simulink model "EDS_Simulink_Model_02"  (R2022a)
settings: Solver=VariableStepAuto  StartTime=0.0  StopTime=stop_time  MaxStep=1e-5  RelTol=1e-3
values from neighbouring files (symbols this model uses):
  a = a/180*pi    [EDS_Script_Model_01.m]    (also in EDS_Script_Model_02.m)
  accel = wheel_radps/accel_time    [EDS_Script_Model_01.m]    (also in EDS_Script_Model_02.m)
  accel_time = 5.33    [EDS_Script_Model_01.m]    (also in EDS_Script_Model_02.m)
  Cx = 0.25    [EDS_Script_Model_01.m]    (also in EDS_Script_Model_02.m)
  d = 1.5    [EDS_Script_Model_01.m]    (also in EDS_Script_Model_02.m)
  density = 1.3    [EDS_Script_Model_01.m]    (also in EDS_Script_Model_02.m)
  F = 4e-04    (= 0.0004)    [EDS_Script_Model_02.m]
  Filter_coefficient = 100/50    (= 2)    [EDS_Script_Model_02.m]
  fr = 0.01    [EDS_Script_Model_01.m]    (also in EDS_Script_Model_02.m)
  g = 9.81    [EDS_Script_Model_01.m]    (also in EDS_Script_Model_02.m)
  i_gear = 7.2    [EDS_Script_Model_01.m]    (also in EDS_Script_Model_02.m = 1)
  J = 0.07/4    (= 0.0175)    [EDS_Script_Model_02.m]
  K_tor_all_1 = 1/2    (= 0.5)    [EDS_Script_Model_01.m]    (also in EDS_Script_Model_02.m)
  K_tor_all_2 = 1/2    (= 0.5)    [EDS_Script_Model_01.m]    (also in EDS_Script_Model_02.m)
  Kd_w = 0.5/8    (= 0.0625)    [EDS_Script_Model_02.m]
  Ki_id = 0.2/14    (= 0.0142857142857)    [EDS_Script_Model_02.m]
  Ki_iq = 10/14    (= 0.714285714286)    [EDS_Script_Model_02.m]
  Ki_w = 2/0.024    (= 83.3333333333)    [EDS_Script_Model_02.m]
  Kp_id = 5/12    (= 0.416666666667)    [EDS_Script_Model_02.m]
  Kp_iq = 30/12    (= 2.5)    [EDS_Script_Model_02.m]
  Kp_w = 55/0.024    (= 2291.66666667)    [EDS_Script_Model_02.m]
  L = 2.5    [EDS_Script_Model_01.m]    (also in EDS_Script_Model_02.m)
  M = 1200    [EDS_Script_Model_01.m]    (also in EDS_Script_Model_02.m)
  n_eff_gear = 0.98    [EDS_Script_Model_01.m]    (also in EDS_Script_Model_02.m = 1)
  p = 4    [EDS_Script_Model_02.m]
  Rs = 4.47-1.47-0.40    (= 2.6)    [EDS_Script_Model_02.m]
  Rw = 0.26    [EDS_Script_Model_01.m]    (also in EDS_Script_Model_02.m)
  S = 1.9    [EDS_Script_Model_01.m]    (also in EDS_Script_Model_02.m)
  Satur_max_PI_id = Vdc_1*sqrt(1/3)    [EDS_Script_Model_02.m]
  Satur_max_PI_iq = Vdc_1*sqrt(1/3)    [EDS_Script_Model_02.m]
  Satur_max_PI_w = 40+30    (= 70)    [EDS_Script_Model_02.m]
  Satur_min_PI_id = -Vdc_1*sqrt(1/3)    [EDS_Script_Model_02.m]
  Satur_min_PI_iq = -Vdc_1*sqrt(1/3)    [EDS_Script_Model_02.m]
  Satur_min_PI_w = -40-30    (= -70)    [EDS_Script_Model_02.m]
  steering_angle_1 = steering_angle_1_m(ii)    [EDS_Script_Model_01.m]    (also in EDS_Script_Model_02.m)
  steering_angle_2 = steering_angle_2_m(ii)    [EDS_Script_Model_01.m]    (also in EDS_Script_Model_02.m)
  steering_angle_3 = steering_angle_3_m(ii)    [EDS_Script_Model_01.m]    (also in EDS_Script_Model_02.m)
  steering_angle_4 = steering_angle_4_m(ii)    [EDS_Script_Model_01.m]    (also in EDS_Script_Model_02.m)
  steering_angle_initial = steering_angle_initial_m(ii)    [EDS_Script_Model_01.m]    (also in EDS_Script_Model_02.m)
  Tf = 0    [EDS_Script_Model_02.m]
  time_steering_angle_1 = 8    [EDS_Script_Model_01.m]    (also in EDS_Script_Model_02.m)
  time_steering_angle_2 = 10    [EDS_Script_Model_01.m]    (also in EDS_Script_Model_02.m)
  time_steering_angle_3 = 14    [EDS_Script_Model_01.m]    (also in EDS_Script_Model_02.m)
  time_steering_angle_4 = 18    [EDS_Script_Model_01.m]    (also in EDS_Script_Model_02.m)
  Vdc_1 = 500    [EDS_Script_Model_02.m]
  Vdc_2 = 500    [EDS_Script_Model_02.m]
  Vf = 0    [EDS_Script_Model_02.m]
  Vfd = 0    [EDS_Script_Model_02.m]
undefined symbols (not defined in the file or in its folder): time_w_ref_1, time_w_ref_2, w_ref_1, w_ref_2, w_ref_initial
libraries: slpidlib x6, spsPermanentMagnetSynchronousMachineLib x2, spsThreePhaseVIMeasurementLib x2, spsUniversalBridgeLib x2, spsDCVoltageSourceLib x2, spsVoltageMeasurementLib x2, spspowerguiLib x1
(part 1 of 2)
settings Model: Creator=panos  LastModifiedBy=panos
settings SolverCC: ConsecutiveZCsStepRelTol=128*eps  MaxConsecutiveZCs=5000
settings DataIOCC: MaxDataPoints=5e5  Refine=4
settings DebuggingCC: IgnoredZcDiagnostic=none

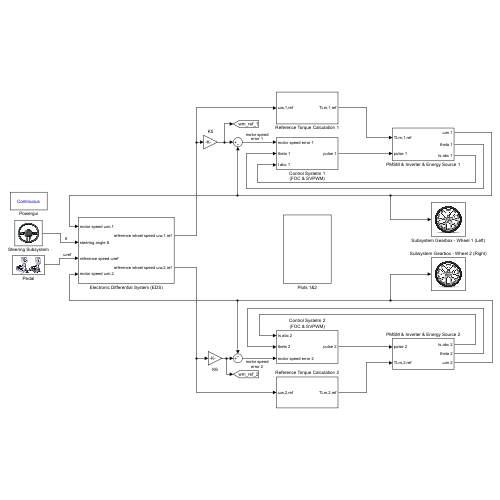
[thumbnail: Simulink's stored preview of the top-level diagram]
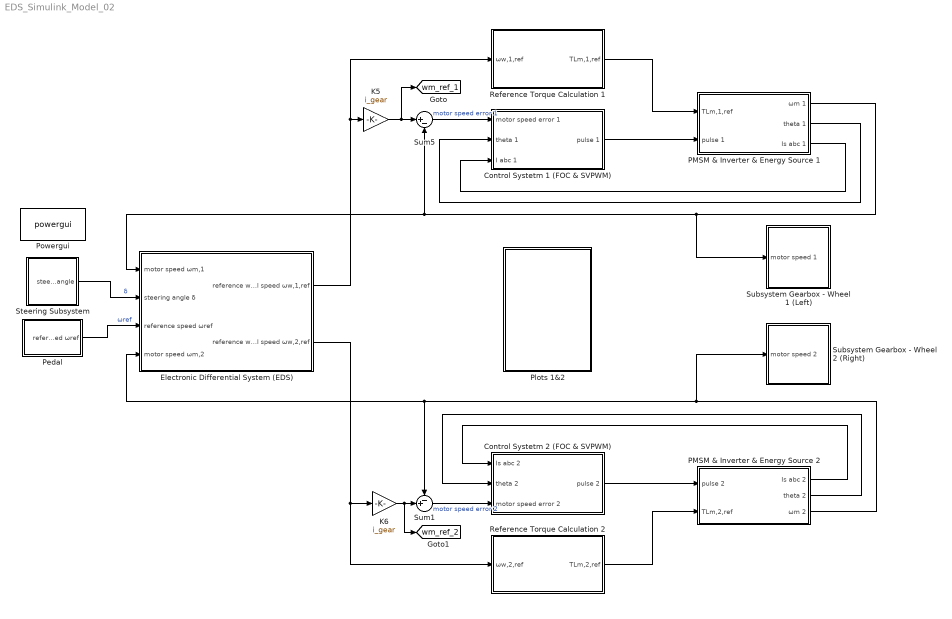
== system EDS_Simulink_Model_02 ==
  Control Systetm 1 (FOC & SVPWM) : Subsystem
  Control Systetm 2 (FOC & SVPWM) : Subsystem
  Electronic Differential System (EDS) : Subsystem
  K5 : Gain  Gain=i_gear
  K6 : Gain  Gain=i_gear
  PMSM & Inverter & Energy Source 1 : Subsystem
  PMSM & Inverter & Energy Source 2 : Subsystem
  Pedal : Subsystem
      mask Display: image('pedal.jpg'); % Use "Edit Image" on toolstrip to change.
  Plots 1&2 : Subsystem
  Powergui : spspowerguiLib/powergui  Priority=1  SimulationMode=Continuous  SampleTime=50e-6  frequency=60  Iterations=50  frequencyindice=0  Pbase=100e6  ErrMax=1e-4  UnitsV=kV  UnitsW=MW  buscounter=0  FunctionMessages=off  echomessages=off  EnableUseOfTLC=off  CurrentSourceSwitches=off  DisableSnubberDevices=off  DisableRonSwitches=off  DisableVfSwitches=off  DisplayEquations=off  AutomaticDiscreteSolvers=off  SolverType=Tustin/Backward Euler (TBE)  Interpol=off  ExternalGateDelay=off  methode=off  Ts=100  x0status=blocks  SPID=on  SwTol=0  HookPort=off  NonlinearTolerance=1e-4  nMaxIteration=100  ContinueOnMaxIteration=off  RestoreLinks=warning  ResistiveCurrentMeasurement=off  Frange=[0:2:500]  Ylog=off  Xlog=on  ShowGrid=off  save=off  variable=ZData  structure=0  ZoomFFT=off  StartTime=0.0  cycles=1  DisplayStyle=1  fundamental=60  FreqAxis=off  MaxFrequency=1000  frequencyindicesteady=1  RmsSteady=1  display=off
  Reference Torque Calculation 1 : Subsystem
  Reference Torque Calculation 2 : Subsystem
  Steering Subsystem : Subsystem
      mask Display: image('steering.jpg'); % Use "Edit Image" on toolstrip to change.
  Subsystem Gearbox - Wheel 1 (Left) : Subsystem
      mask Display: image('C:\Users\panos\OneDrive\Υπολογιστής\Desktop\Master_Thesis\electronic differential system (EDS)\PHOTO\wheel.jpg'); % Use "Edit Image" on toolstrip to change.
  Subsystem Gearbox - Wheel 2 (Right) : Subsystem
      mask Display: image('C:\Users\panos\OneDrive\Υπολογιστής\Desktop\Master_Thesis\electronic differential system (EDS)\PHOTO\wheel.jpg'); % Use "Edit Image" on toolstrip to change.
  Sum1 : Sum  Inputs=-+|
  Sum5 : Sum  Inputs=|+-
  tag scope: wm_ref_1=global, wm_ref_2=global
  wires:
  Sum1/1 -> Control Systetm 2 (FOC & SVPWM)/3(motor speed error 2)  "motor speed error 2"
  PMSM & Inverter & Energy Source 2/3(ωm 2) -> Sum1/1, Electronic Differential System (EDS)/4(motor speed ωm,2), Subsystem Gearbox - Wheel 2 (Right)/1(motor speed 2)
  Sum5/1 -> Control Systetm 1 (FOC & SVPWM)/1(motor speed error 1)  "motor speed error 1"
  PMSM & Inverter & Energy Source 1/1(ωm 1) -> Subsystem Gearbox - Wheel 1 (Left)/1(motor speed 1), Sum5/2, Electronic Differential System (EDS)/1(motor speed ωm,1)
  Electronic Differential System (EDS)/1("reference wheel speed ωw,1,ref ") -> Reference Torque Calculation 1/1(ωw,1,ref), K5/1
  Electronic Differential System (EDS)/2("reference wheel speed ωw,2,ref ") -> Reference Torque Calculation 2/1(ωw,2,ref), K6/1
  Steering Subsystem/1(steering angle) -> Electronic Differential System (EDS)/2(steering angle δ)  "δ"
  Pedal/1(reference speed ωref) -> Electronic Differential System (EDS)/3(reference speed ωref)  "ωref"
  Reference Torque Calculation 1/1(TLm,1,ref) -> PMSM & Inverter & Energy Source 1/1(TLm,1,ref)
  Reference Torque Calculation 2/1(TLm,2,ref) -> PMSM & Inverter & Energy Source 2/2(TLm,2,ref)
  K6/1 -> Sum1/2, [wm_ref_2]
  Control Systetm 2 (FOC & SVPWM)/1(pulse 2) -> PMSM & Inverter & Energy Source 2/1(pulse 2)
  Control Systetm 1 (FOC & SVPWM)/1(pulse 1) -> PMSM & Inverter & Energy Source 1/2(pulse 1)
  PMSM & Inverter & Energy Source 1/2(theta 1) -> Control Systetm 1 (FOC & SVPWM)/2(theta 1)
  PMSM & Inverter & Energy Source 1/3(Is abc 1) -> Control Systetm 1 (FOC & SVPWM)/3(I abc 1)
  K5/1 -> [wm_ref_1], Sum5/1
  PMSM & Inverter & Energy Source 2/2(theta 2) -> Control Systetm 2 (FOC & SVPWM)/2(theta 2)
  PMSM & Inverter & Energy Source 2/1(Is abc 2) -> Control Systetm 2 (FOC & SVPWM)/1(Is abc 2)

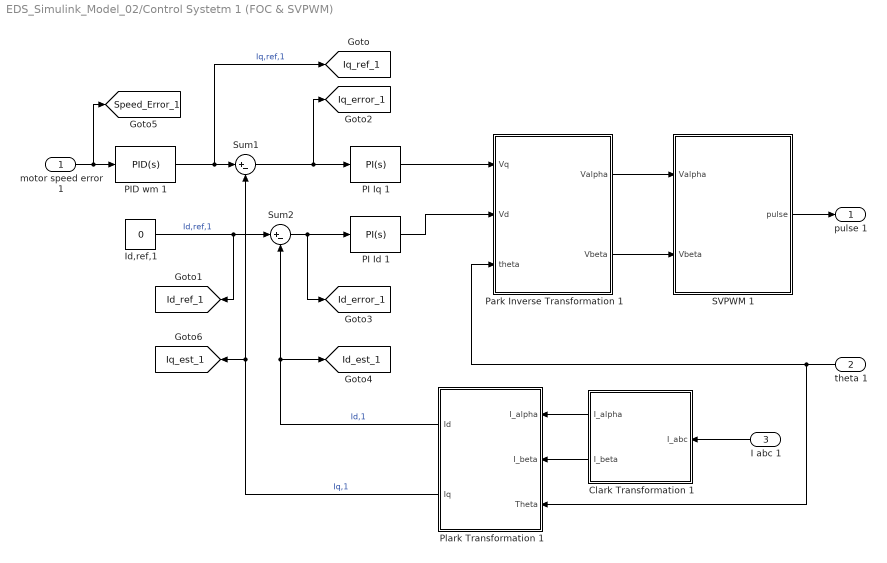
== system EDS_Simulink_Model_02/Control Systetm 1 (FOC & SVPWM) ==
  motor speed error 1 : Inport
  theta 1 : Inport  Port=2
  I abc 1 : Inport  Port=3
  Clark Transformation 1 : Subsystem
  Id,ref,1 : Constant  Value=0
  "PI Id 1 " : slpidlib/PID Controller  Controller=PI  Form=Parallel  TimeDomain=Continuous-time  UseExternalTs=off  SampleTime=-1  IntegratorMethod=Forward Euler  FilterMethod=Forward Euler  ControllerParametersSource=internal  P=Kp_id  I=Ki_id  UseKiTs=off  D=0  N=100  UseFilter=on  TunerSelectOption=Transfer Function Based (PID Tuner App)  InitialConditionSource=internal  InitialConditionForIntegrator=0  InitialConditionForFilter=0  DifferentiatorICPrevScaledInput=0  ExternalReset=none  TrackingMode=off  Kt=1  LimitOutput=on  SatLimitsSource=internal  UpperSaturationLimit=Satur_max_PI_id  LowerSaturationLimit=Satur_min_PI_id  LinearizeAsGain=on  AntiWindupMode=none  Kb=1  POutMin=[]  POutMax=[]  IOutMin=[]  IOutMax=[]  DOutMin=[]  DOutMax=[]  NOutMin=[]  NOutMax=[]  SumOutMin=[]  SumOutMax=[]  SaturationOutMin=[]  SaturationOutMax=[]  PParamMin=[]  PParamMax=[]  IParamMin=[]  IParamMax=[]  DParamMin=[]  DParamMax=[]  NParamMin=[]  NParamMax=[]  KbParamMin=[]  KbParamMax=[]  KtParamMin=[]  KtParamMax=[]  KbOutMin=[]  KbOutMax=[]  KtOutMin=[]  KtOutMax=[]  IntegratorOutMin=[]  IntegratorOutMax=[]  FilterOutMin=[]  FilterOutMax=[]  SumI1OutMin=[]  SumI1OutMax=[]  SumI2OutMin=[]  SumI2OutMax=[]  SumI3OutMin=[]  SumI3OutMax=[]  SumI4OutMin=[]  SumI4OutMax=[]  SumDOutMin=[]  SumDOutMax=[]  DifferentiatorOutMin=[]  DifferentiatorOutMax=[]  FilterDiffOutCoefMin=[]  FilterDiffOutCoefMax=[]  ReciprocalOutMin=[]  ReciprocalOutMax=[]  SumDenOutMin=[]  SumDenOutMax=[]  SumNumOutMin=[]  SumNumOutMax=[]  DivideOutMin=[]  DivideOutMax=[]  UdiffTsProdOutMin=[]  UdiffTsProdOutMax=[]  NTsProdOutMin=[]  NTsProdOutMax=[]  UintegralTsProdOutMin=[]  UintegralTsProdOutMax=[]  UngainTsProdOutMin=[]  UngainTsProdOutMax=[]  IntegratorContinuousStateAttributes=''  IntegratorStateMustResolveToSignalObject=off  IntegratorRTWStateStorageClass=Auto  FilterContinuousStateAttributes=''  FilterStateMustResolveToSignalObject=off  FilterRTWStateStorageClass=Auto  ParallelPVariant=InternalParameters  IdealPVariant=Disabled  IVariant=InternalParameters  DVariant=Disabled  IntegratorVariant=Continuous  SatVariant=Enabled  AWVariant=Passthrough  PCopyVariant=Disabled  TRVariant=Disabled  FdbkBlocksVariant=Forward  IdealPFdbkVariant=Disabled  SatFdbkVariant=Disabled  DerivativeFilterVariant=Disabled  NVariant=Disabled  NCopyVariant=Disabled_SignalSpec  FilterICVariant=Disabled  IntegratorICVariant=InternalICs  ExternalResetVariant=Disabled  TRSumVariant=Passthrough  SumFdbkVariant=Disabled  SumVariant=Sum_PI  TsampFilterVariant=InternalTs  TsampNgainVariant=Passthrough  TsampIntegralVariant=Passthrough  ExternalSaturationOutDataTypeStr=Inherit: Same as second input  aMode=0
  PI Iq 1 : slpidlib/PID Controller  Controller=PI  Form=Parallel  TimeDomain=Continuous-time  UseExternalTs=off  SampleTime=-1  IntegratorMethod=Forward Euler  FilterMethod=Forward Euler  ControllerParametersSource=internal  P=Kp_iq  I=Ki_iq  UseKiTs=off  D=0  N=100  UseFilter=on  TunerSelectOption=Transfer Function Based (PID Tuner App)  InitialConditionSource=internal  InitialConditionForIntegrator=0  InitialConditionForFilter=0  DifferentiatorICPrevScaledInput=0  ExternalReset=none  TrackingMode=off  Kt=1  LimitOutput=on  SatLimitsSource=internal  UpperSaturationLimit=Satur_max_PI_iq  LowerSaturationLimit=Satur_min_PI_iq  LinearizeAsGain=on  AntiWindupMode=none  Kb=1  POutMin=[]  POutMax=[]  IOutMin=[]  IOutMax=[]  DOutMin=[]  DOutMax=[]  NOutMin=[]  NOutMax=[]  SumOutMin=[]  SumOutMax=[]  SaturationOutMin=[]  SaturationOutMax=[]  PParamMin=[]  PParamMax=[]  IParamMin=[]  IParamMax=[]  DParamMin=[]  DParamMax=[]  NParamMin=[]  NParamMax=[]  KbParamMin=[]  KbParamMax=[]  KtParamMin=[]  KtParamMax=[]  KbOutMin=[]  KbOutMax=[]  KtOutMin=[]  KtOutMax=[]  IntegratorOutMin=[]  IntegratorOutMax=[]  FilterOutMin=[]  FilterOutMax=[]  SumI1OutMin=[]  SumI1OutMax=[]  SumI2OutMin=[]  SumI2OutMax=[]  SumI3OutMin=[]  SumI3OutMax=[]  SumI4OutMin=[]  SumI4OutMax=[]  SumDOutMin=[]  SumDOutMax=[]  DifferentiatorOutMin=[]  DifferentiatorOutMax=[]  FilterDiffOutCoefMin=[]  FilterDiffOutCoefMax=[]  ReciprocalOutMin=[]  ReciprocalOutMax=[]  SumDenOutMin=[]  SumDenOutMax=[]  SumNumOutMin=[]  SumNumOutMax=[]  DivideOutMin=[]  DivideOutMax=[]  UdiffTsProdOutMin=[]  UdiffTsProdOutMax=[]  NTsProdOutMin=[]  NTsProdOutMax=[]  UintegralTsProdOutMin=[]  UintegralTsProdOutMax=[]  UngainTsProdOutMin=[]  UngainTsProdOutMax=[]  IntegratorContinuousStateAttributes=''  IntegratorStateMustResolveToSignalObject=off  IntegratorRTWStateStorageClass=Auto  FilterContinuousStateAttributes=''  FilterStateMustResolveToSignalObject=off  FilterRTWStateStorageClass=Auto  ParallelPVariant=InternalParameters  IdealPVariant=Disabled  IVariant=InternalParameters  DVariant=Disabled  IntegratorVariant=Continuous  SatVariant=Enabled  AWVariant=Passthrough  PCopyVariant=Disabled  TRVariant=Disabled  FdbkBlocksVariant=Forward  IdealPFdbkVariant=Disabled  SatFdbkVariant=Disabled  DerivativeFilterVariant=Disabled  NVariant=Disabled  NCopyVariant=Disabled_SignalSpec  FilterICVariant=Disabled  IntegratorICVariant=InternalICs  ExternalResetVariant=Disabled  TRSumVariant=Passthrough  SumFdbkVariant=Disabled  SumVariant=Sum_PI  TsampFilterVariant=InternalTs  TsampNgainVariant=Passthrough  TsampIntegralVariant=Passthrough  ExternalSaturationOutDataTypeStr=Inherit: Same as second input  aMode=0
  PID wm 1 : slpidlib/PID Controller  Controller=PID  Form=Parallel  TimeDomain=Continuous-time  UseExternalTs=off  SampleTime=-1  IntegratorMethod=Forward Euler  FilterMethod=Forward Euler  ControllerParametersSource=internal  P=Kp_w  I=Ki_w  UseKiTs=off  D=Kd_w  N=Filter_coefficient  UseFilter=on  TunerSelectOption=Transfer Function Based (PID Tuner App)  InitialConditionSource=internal  InitialConditionForIntegrator=0  InitialConditionForFilter=0  DifferentiatorICPrevScaledInput=0  ExternalReset=none  TrackingMode=off  Kt=1  LimitOutput=on  SatLimitsSource=internal  UpperSaturationLimit=Satur_max_PI_w  LowerSaturationLimit=Satur_min_PI_w  LinearizeAsGain=on  AntiWindupMode=none  Kb=1  POutMin=[]  POutMax=[]  IOutMin=[]  IOutMax=[]  DOutMin=[]  DOutMax=[]  NOutMin=[]  NOutMax=[]  SumOutMin=[]  SumOutMax=[]  SaturationOutMin=[]  SaturationOutMax=[]  PParamMin=[]  PParamMax=[]  IParamMin=[]  IParamMax=[]  DParamMin=[]  DParamMax=[]  NParamMin=[]  NParamMax=[]  KbParamMin=[]  KbParamMax=[]  KtParamMin=[]  KtParamMax=[]  KbOutMin=[]  KbOutMax=[]  KtOutMin=[]  KtOutMax=[]  IntegratorOutMin=[]  IntegratorOutMax=[]  FilterOutMin=[]  FilterOutMax=[]  SumI1OutMin=[]  SumI1OutMax=[]  SumI2OutMin=[]  SumI2OutMax=[]  SumI3OutMin=[]  SumI3OutMax=[]  SumI4OutMin=[]  SumI4OutMax=[]  SumDOutMin=[]  SumDOutMax=[]  DifferentiatorOutMin=[]  DifferentiatorOutMax=[]  FilterDiffOutCoefMin=[]  FilterDiffOutCoefMax=[]  ReciprocalOutMin=[]  ReciprocalOutMax=[]  SumDenOutMin=[]  SumDenOutMax=[]  SumNumOutMin=[]  SumNumOutMax=[]  DivideOutMin=[]  DivideOutMax=[]  UdiffTsProdOutMin=[]  UdiffTsProdOutMax=[]  NTsProdOutMin=[]  NTsProdOutMax=[]  UintegralTsProdOutMin=[]  UintegralTsProdOutMax=[]  UngainTsProdOutMin=[]  UngainTsProdOutMax=[]  IntegratorContinuousStateAttributes=''  IntegratorStateMustResolveToSignalObject=off  IntegratorRTWStateStorageClass=Auto  FilterContinuousStateAttributes=''  FilterStateMustResolveToSignalObject=off  FilterRTWStateStorageClass=Auto  ParallelPVariant=InternalParameters  IdealPVariant=Disabled  IVariant=InternalParameters  DVariant=InternalParameters  IntegratorVariant=Continuous  SatVariant=Enabled  AWVariant=Passthrough  PCopyVariant=Disabled  TRVariant=Disabled  FdbkBlocksVariant=Forward  IdealPFdbkVariant=Disabled  SatFdbkVariant=Disabled  DerivativeFilterVariant=ContFilter  NVariant=InternalParameters  NCopyVariant=Disabled  FilterICVariant=InternalICsFilter  IntegratorICVariant=InternalICs  ExternalResetVariant=Disabled  TRSumVariant=Passthrough  SumFdbkVariant=Disabled  SumVariant=Sum_PID  TsampFilterVariant=InternalTs  TsampNgainVariant=Passthrough  TsampIntegralVariant=Passthrough  ExternalSaturationOutDataTypeStr=Inherit: Same as second input  aMode=0
  "Park Inverse Transformation 1 " : Subsystem
  Plark Transformation 1 : Subsystem
  SVPWM 1 : Subsystem
  Sum1 : Sum  Inputs=|+-
  Sum2 : Sum  Inputs=|+-
  pulse 1 : Outport
  tag scope: Id_error_1=global, Id_est_1=global, Id_ref_1=global, Iq_error_1=global, Iq_est_1=global, Iq_ref_1=global, Speed_Error_1=global
  wires:
  PI Iq 1/1 -> "Park Inverse Transformation 1 "/1(Vq)
  PID wm 1/1 -> [Iq_ref_1], Sum1/1  "Iq,ref,1"
  "PI Id 1 "/1 -> "Park Inverse Transformation 1 "/2(Vd)
  Id,ref,1/1 -> Sum2/1, [Id_ref_1]  "Id,ref,1"
  Plark Transformation 1/2(Iq) -> [Iq_est_1], Sum1/2  "Iq,1"
  "Park Inverse Transformation 1 "/2(Vbeta) -> SVPWM 1/2(Vbeta)
  Clark Transformation 1/2(I_beta) -> Plark Transformation 1/2(I_beta)
  Plark Transformation 1/1(Id) -> Sum2/2, [Id_est_1]  "Id,1"
  Sum2/1 -> [Id_error_1], "PI Id 1 "/1
  theta 1/1 -> Plark Transformation 1/3(Theta), "Park Inverse Transformation 1 "/3(theta)
  "Park Inverse Transformation 1 "/1(Valpha) -> SVPWM 1/1(Valpha)
  I abc 1/1 -> Clark Transformation 1/1(I_abc)
  SVPWM 1/1(pulse) -> pulse 1/1
  Sum1/1 -> PI Iq 1/1, [Iq_error_1]
  motor speed error 1/1 -> PID wm 1/1, [Speed_Error_1]
  Clark Transformation 1/1(I_alpha) -> Plark Transformation 1/1(I_alpha)

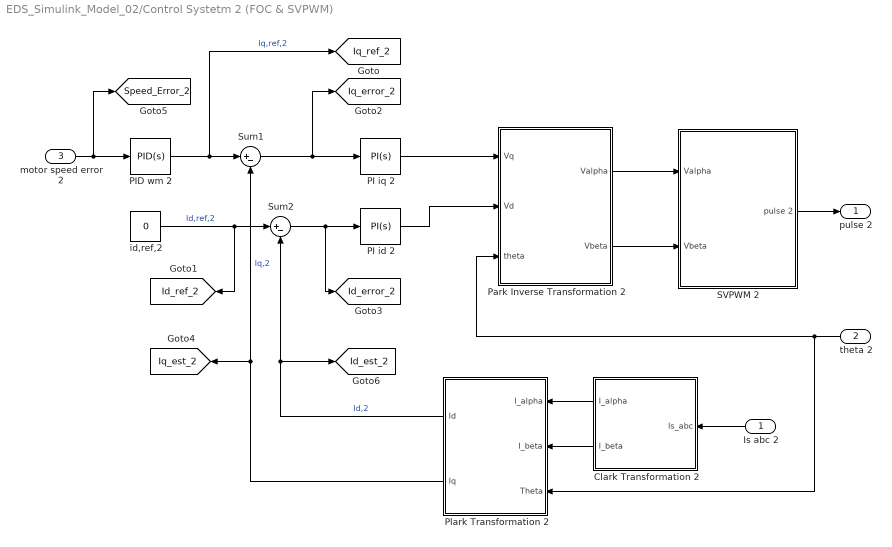
== system EDS_Simulink_Model_02/Control Systetm 2 (FOC & SVPWM) ==
  Is abc 2 : Inport
  theta 2 : Inport  Port=2
  motor speed error 2 : Inport  Port=3
  Clark Transformation 2 : Subsystem
  "PI id 2 " : slpidlib/PID Controller  Controller=PI  Form=Parallel  TimeDomain=Continuous-time  UseExternalTs=off  SampleTime=-1  IntegratorMethod=Forward Euler  FilterMethod=Forward Euler  ControllerParametersSource=internal  P=Kp_id  I=Ki_id  UseKiTs=off  D=0  N=100  UseFilter=on  TunerSelectOption=Transfer Function Based (PID Tuner App)  InitialConditionSource=internal  InitialConditionForIntegrator=0  InitialConditionForFilter=0  DifferentiatorICPrevScaledInput=0  ExternalReset=none  TrackingMode=off  Kt=1  LimitOutput=on  SatLimitsSource=internal  UpperSaturationLimit=Satur_max_PI_id  LowerSaturationLimit=Satur_min_PI_id  LinearizeAsGain=on  AntiWindupMode=none  Kb=1  POutMin=[]  POutMax=[]  IOutMin=[]  IOutMax=[]  DOutMin=[]  DOutMax=[]  NOutMin=[]  NOutMax=[]  SumOutMin=[]  SumOutMax=[]  SaturationOutMin=[]  SaturationOutMax=[]  PParamMin=[]  PParamMax=[]  IParamMin=[]  IParamMax=[]  DParamMin=[]  DParamMax=[]  NParamMin=[]  NParamMax=[]  KbParamMin=[]  KbParamMax=[]  KtParamMin=[]  KtParamMax=[]  KbOutMin=[]  KbOutMax=[]  KtOutMin=[]  KtOutMax=[]  IntegratorOutMin=[]  IntegratorOutMax=[]  FilterOutMin=[]  FilterOutMax=[]  SumI1OutMin=[]  SumI1OutMax=[]  SumI2OutMin=[]  SumI2OutMax=[]  SumI3OutMin=[]  SumI3OutMax=[]  SumI4OutMin=[]  SumI4OutMax=[]  SumDOutMin=[]  SumDOutMax=[]  DifferentiatorOutMin=[]  DifferentiatorOutMax=[]  FilterDiffOutCoefMin=[]  FilterDiffOutCoefMax=[]  ReciprocalOutMin=[]  ReciprocalOutMax=[]  SumDenOutMin=[]  SumDenOutMax=[]  SumNumOutMin=[]  SumNumOutMax=[]  DivideOutMin=[]  DivideOutMax=[]  UdiffTsProdOutMin=[]  UdiffTsProdOutMax=[]  NTsProdOutMin=[]  NTsProdOutMax=[]  UintegralTsProdOutMin=[]  UintegralTsProdOutMax=[]  UngainTsProdOutMin=[]  UngainTsProdOutMax=[]  IntegratorContinuousStateAttributes=''  IntegratorStateMustResolveToSignalObject=off  IntegratorRTWStateStorageClass=Auto  FilterContinuousStateAttributes=''  FilterStateMustResolveToSignalObject=off  FilterRTWStateStorageClass=Auto  ParallelPVariant=InternalParameters  IdealPVariant=Disabled  IVariant=InternalParameters  DVariant=Disabled  IntegratorVariant=Continuous  SatVariant=Enabled  AWVariant=Passthrough  PCopyVariant=Disabled  TRVariant=Disabled  FdbkBlocksVariant=Forward  IdealPFdbkVariant=Disabled  SatFdbkVariant=Disabled  DerivativeFilterVariant=Disabled  NVariant=Disabled  NCopyVariant=Disabled_SignalSpec  FilterICVariant=Disabled  IntegratorICVariant=InternalICs  ExternalResetVariant=Disabled  TRSumVariant=Passthrough  SumFdbkVariant=Disabled  SumVariant=Sum_PI  TsampFilterVariant=InternalTs  TsampNgainVariant=Passthrough  TsampIntegralVariant=Passthrough  ExternalSaturationOutDataTypeStr=Inherit: Same as second input  aMode=0
  PI iq 2 : slpidlib/PID Controller  Controller=PI  Form=Parallel  TimeDomain=Continuous-time  UseExternalTs=off  SampleTime=-1  IntegratorMethod=Forward Euler  FilterMethod=Forward Euler  ControllerParametersSource=internal  P=Kp_iq  I=Ki_iq  UseKiTs=off  D=0  N=100  UseFilter=on  TunerSelectOption=Transfer Function Based (PID Tuner App)  InitialConditionSource=internal  InitialConditionForIntegrator=0  InitialConditionForFilter=0  DifferentiatorICPrevScaledInput=0  ExternalReset=none  TrackingMode=off  Kt=1  LimitOutput=on  SatLimitsSource=internal  UpperSaturationLimit=Satur_max_PI_iq  LowerSaturationLimit=Satur_min_PI_iq  LinearizeAsGain=on  AntiWindupMode=none  Kb=1  POutMin=[]  POutMax=[]  IOutMin=[]  IOutMax=[]  DOutMin=[]  DOutMax=[]  NOutMin=[]  NOutMax=[]  SumOutMin=[]  SumOutMax=[]  SaturationOutMin=[]  SaturationOutMax=[]  PParamMin=[]  PParamMax=[]  IParamMin=[]  IParamMax=[]  DParamMin=[]  DParamMax=[]  NParamMin=[]  NParamMax=[]  KbParamMin=[]  KbParamMax=[]  KtParamMin=[]  KtParamMax=[]  KbOutMin=[]  KbOutMax=[]  KtOutMin=[]  KtOutMax=[]  IntegratorOutMin=[]  IntegratorOutMax=[]  FilterOutMin=[]  FilterOutMax=[]  SumI1OutMin=[]  SumI1OutMax=[]  SumI2OutMin=[]  SumI2OutMax=[]  SumI3OutMin=[]  SumI3OutMax=[]  SumI4OutMin=[]  SumI4OutMax=[]  SumDOutMin=[]  SumDOutMax=[]  DifferentiatorOutMin=[]  DifferentiatorOutMax=[]  FilterDiffOutCoefMin=[]  FilterDiffOutCoefMax=[]  ReciprocalOutMin=[]  ReciprocalOutMax=[]  SumDenOutMin=[]  SumDenOutMax=[]  SumNumOutMin=[]  SumNumOutMax=[]  DivideOutMin=[]  DivideOutMax=[]  UdiffTsProdOutMin=[]  UdiffTsProdOutMax=[]  NTsProdOutMin=[]  NTsProdOutMax=[]  UintegralTsProdOutMin=[]  UintegralTsProdOutMax=[]  UngainTsProdOutMin=[]  UngainTsProdOutMax=[]  IntegratorContinuousStateAttributes=''  IntegratorStateMustResolveToSignalObject=off  IntegratorRTWStateStorageClass=Auto  FilterContinuousStateAttributes=''  FilterStateMustResolveToSignalObject=off  FilterRTWStateStorageClass=Auto  ParallelPVariant=InternalParameters  IdealPVariant=Disabled  IVariant=InternalParameters  DVariant=Disabled  IntegratorVariant=Continuous  SatVariant=Enabled  AWVariant=Passthrough  PCopyVariant=Disabled  TRVariant=Disabled  FdbkBlocksVariant=Forward  IdealPFdbkVariant=Disabled  SatFdbkVariant=Disabled  DerivativeFilterVariant=Disabled  NVariant=Disabled  NCopyVariant=Disabled_SignalSpec  FilterICVariant=Disabled  IntegratorICVariant=InternalICs  ExternalResetVariant=Disabled  TRSumVariant=Passthrough  SumFdbkVariant=Disabled  SumVariant=Sum_PI  TsampFilterVariant=InternalTs  TsampNgainVariant=Passthrough  TsampIntegralVariant=Passthrough  ExternalSaturationOutDataTypeStr=Inherit: Same as second input  aMode=0
  PID wm 2 : slpidlib/PID Controller  Controller=PID  Form=Parallel  TimeDomain=Continuous-time  UseExternalTs=off  SampleTime=-1  IntegratorMethod=Forward Euler  FilterMethod=Forward Euler  ControllerParametersSource=internal  P=Kp_w  I=Ki_w  UseKiTs=off  D=Kd_w  N=Filter_coefficient  UseFilter=on  TunerSelectOption=Transfer Function Based (PID Tuner App)  InitialConditionSource=internal  InitialConditionForIntegrator=0  InitialConditionForFilter=0  DifferentiatorICPrevScaledInput=0  ExternalReset=none  TrackingMode=off  Kt=1  LimitOutput=on  SatLimitsSource=internal  UpperSaturationLimit=Satur_max_PI_w  LowerSaturationLimit=Satur_min_PI_w  LinearizeAsGain=on  AntiWindupMode=none  Kb=1  POutMin=[]  POutMax=[]  IOutMin=[]  IOutMax=[]  DOutMin=[]  DOutMax=[]  NOutMin=[]  NOutMax=[]  SumOutMin=[]  SumOutMax=[]  SaturationOutMin=[]  SaturationOutMax=[]  PParamMin=[]  PParamMax=[]  IParamMin=[]  IParamMax=[]  DParamMin=[]  DParamMax=[]  NParamMin=[]  NParamMax=[]  KbParamMin=[]  KbParamMax=[]  KtParamMin=[]  KtParamMax=[]  KbOutMin=[]  KbOutMax=[]  KtOutMin=[]  KtOutMax=[]  IntegratorOutMin=[]  IntegratorOutMax=[]  FilterOutMin=[]  FilterOutMax=[]  SumI1OutMin=[]  SumI1OutMax=[]  SumI2OutMin=[]  SumI2OutMax=[]  SumI3OutMin=[]  SumI3OutMax=[]  SumI4OutMin=[]  SumI4OutMax=[]  SumDOutMin=[]  SumDOutMax=[]  DifferentiatorOutMin=[]  DifferentiatorOutMax=[]  FilterDiffOutCoefMin=[]  FilterDiffOutCoefMax=[]  ReciprocalOutMin=[]  ReciprocalOutMax=[]  SumDenOutMin=[]  SumDenOutMax=[]  SumNumOutMin=[]  SumNumOutMax=[]  DivideOutMin=[]  DivideOutMax=[]  UdiffTsProdOutMin=[]  UdiffTsProdOutMax=[]  NTsProdOutMin=[]  NTsProdOutMax=[]  UintegralTsProdOutMin=[]  UintegralTsProdOutMax=[]  UngainTsProdOutMin=[]  UngainTsProdOutMax=[]  IntegratorContinuousStateAttributes=''  IntegratorStateMustResolveToSignalObject=off  IntegratorRTWStateStorageClass=Auto  FilterContinuousStateAttributes=''  FilterStateMustResolveToSignalObject=off  FilterRTWStateStorageClass=Auto  ParallelPVariant=InternalParameters  IdealPVariant=Disabled  IVariant=InternalParameters  DVariant=InternalParameters  IntegratorVariant=Continuous  SatVariant=Enabled  AWVariant=Passthrough  PCopyVariant=Disabled  TRVariant=Disabled  FdbkBlocksVariant=Forward  IdealPFdbkVariant=Disabled  SatFdbkVariant=Disabled  DerivativeFilterVariant=ContFilter  NVariant=InternalParameters  NCopyVariant=Disabled  FilterICVariant=InternalICsFilter  IntegratorICVariant=InternalICs  ExternalResetVariant=Disabled  TRSumVariant=Passthrough  SumFdbkVariant=Disabled  SumVariant=Sum_PID  TsampFilterVariant=InternalTs  TsampNgainVariant=Passthrough  TsampIntegralVariant=Passthrough  ExternalSaturationOutDataTypeStr=Inherit: Same as second input  aMode=0
  "Park Inverse Transformation 2 " : Subsystem
  Plark Transformation 2 : Subsystem
  SVPWM 2 : Subsystem
  Sum1 : Sum  Inputs=|+-
  Sum2 : Sum  Inputs=|+-
  id,ref,2 : Constant  Value=0
  pulse 2 : Outport
  tag scope: Id_error_2=global, Id_est_2=global, Id_ref_2=global, Iq_error_2=global, Iq_est_2=global, Iq_ref_2=global, Speed_Error_2=global
  wires:
  PI iq 2/1 -> "Park Inverse Transformation 2 "/1(Vq)
  PID wm 2/1 -> Sum1/1, [Iq_ref_2]  "Iq,ref,2"
  "PI id 2 "/1 -> "Park Inverse Transformation 2 "/2(Vd)
  id,ref,2/1 -> Sum2/1, [Id_ref_2]  "Id,ref,2"
  Plark Transformation 2/2(Iq) -> Sum1/2, [Iq_est_2]  "Iq,2"
  "Park Inverse Transformation 2 "/2(Vbeta) -> SVPWM 2/2(Vbeta)
  Plark Transformation 2/1(Id) -> Sum2/2, [Id_est_2]  "Id,2"
  Sum2/1 -> [Id_error_2], "PI id 2 "/1
  theta 2/1 -> Plark Transformation 2/3(Theta), "Park Inverse Transformation 2 "/3(theta)
  "Park Inverse Transformation 2 "/1(Valpha) -> SVPWM 2/1(Valpha)
  SVPWM 2/1(pulse 2) -> pulse 2/1
  Sum1/1 -> [Iq_error_2], PI iq 2/1
  motor speed error 2/1 -> PID wm 2/1, [Speed_Error_2]
  Is abc 2/1 -> Clark Transformation 2/1(Is_abc)
  Clark Transformation 2/1(I_alpha) -> Plark Transformation 2/1(I_alpha)
  Clark Transformation 2/2(I_beta) -> Plark Transformation 2/2(I_beta)

== system EDS_Simulink_Model_02/Electronic Differential System (EDS) ==
  motor speed ωm,1 : Inport
  steering angle δ : Inport  Port=2
  reference speed ωref : Inport  Port=3
  motor speed ωm,2 : Inport  Port=4
  K1 : Gain  Gain=-1/2
  K2 : Gain  Gain=1/2
  K3 : Gain  Gain=1/i_gear
  K4 : Gain  Gain=1/i_gear
  Sum1 : Sum  Inputs=|-+
  Sum2 : Sum  Inputs=+-|
  center of turn angular speed ωv calculation : MATLAB Function  TreatAsAtomicUnit=on
  difference speed Δω calculation : MATLAB Function  TreatAsAtomicUnit=on
  "reference wheel speed ωw,1,ref " : Outport
  "reference wheel speed ωw,2,ref " : Outport  Port=2
  tag scope: Center_of_turn_Angular_Speed=global, Difference_Speed=global
  wires:
  motor speed ωm,1/1 -> K3/1  "motor speed ωm,1"
  motor speed ωm,2/1 -> K4/1  "motor speed ωm,2"
  K2/1 -> Sum2/2  "Κ2 Δω"
  K1/1 -> Sum1/1  "Κ1 Δω"
  Sum2/1 -> "reference wheel speed ωw,2,ref "/1  "ref wheel speed ωw,2,ref"
  center of turn angular speed ωv calculation/1(wv) -> difference speed Δω calculation/2(wv), [Center_of_turn_Angular_Speed]  "center of turn angular speed ωv"
  difference speed Δω calculation/1(dw) -> [Difference_Speed], K2/1, K1/1  "Δω"
  steering angle δ/1 -> difference speed Δω calculation/1(delta)
  K3/1 -> center of turn angular speed ωv calculation/1(w1_est)  "wheel speed ωw,1"
  Sum1/1 -> "reference wheel speed ωw,1,ref "/1  "ref wheel speed ωw,1,ref"
  K4/1 -> center of turn angular speed ωv calculation/2(w2_est)  "wheel speed ωw,2"
  reference speed ωref/1 -> Sum2/1, Sum1/2

== system EDS_Simulink_Model_02/PMSM & Inverter & Energy Source 1 ==
  TLm,1,ref : Inport
  pulse 1 : Inport  Port=2
  Bus Creator : BusCreator  Inputs=3
  Bus Selector : BusSelector  OutputSignals=Stator current is_a (A),Stator current is_b (A),Stator current is_c (A),Rotor speed wm (rad/s),Rotor angle thetam (rad)
  Gain : Gain  Gain=p
  Gain1 : Gain  Gain=-1
  Permanent Magnet Synchronous Machine 1 : spsPermanentMagnetSynchronousMachineLib/Permanent Magnet Synchronous Machine  NbPhases=3  FluxDistribution=Sinusoidal  RotorType=Round  MechanicalLoad=Torque Tm  PresetModel=No  ShowDetailedParameters=on  MeasurementBus=off  Resistance=Rs  Inductance=8.5e-3  dqInductances=[0.005173 0.005507]  La=La  MachineConstant=Torque Constant (N.m / A_peak)  Flux=0.46667  VoltageCst=338.5759  TorqueCst=Kt  Flat=120  Mechanical=[J F p Tf]  PolePairs=4  InitialConditions=[0,0, 0,0]  InitialConditions5ph=[0 0 0 0 0 0]  RefAngle=90 degrees behind phase A axis (modified Park)  IterativeDiscreteModel=Trapezoidal non iterative  TsBlock=-1  TsPowergui=0
  Three-Phase V-I Measurement 1 : spsThreePhaseVIMeasurementLib/Three-Phase V-I Measurement  VoltageMeasurement=phase-to-phase  SetLabelV=off  LabelV=Vabc  Vpu=off  VpuLL=off  CurrentMeasurement=yes  SetLabelI=off  LabelI=Iabc  Ipu=off  Pbase=100e6  Vbase=500e3  OutputType=Complex  PhasorSimulation=off  PSBequivalent=0
  Universal Bridge Inverter 1 : spsUniversalBridgeLib/Universal Bridge  Arms=3  SnubberResistance=R_snubber  SnubberCapacitance=Cs  Device=IGBT / Diodes  Ron=Ron  Lon=0  ForwardVoltages="[Vf  Vfd]"  ForwardVoltage=0  GTOparameters=[ 10e-6 , 20e-6 ]  IGBTparameters=[ 1e-6 , 2e-6 ]  Measurements=Device voltages  Measurements_2=None  converterType=Rectifier
  Vdc 1 : spsDCVoltageSourceLib/DC Voltage Source  Amplitude=Vdc_1  Measurements=None
  Voltage Measurement 1 : spsVoltageMeasurementLib/Voltage Measurement  PhasorSimulation=off  OutputType=Complex  PSBequivalent=0
  ωm 1 : Outport  VectorParamsAs1DForOutWhenUnconnected=off
  theta 1 : Outport  Port=2  VectorParamsAs1DForOutWhenUnconnected=off
  Is abc 1 : Outport  Port=3  VectorParamsAs1DForOutWhenUnconnected=off
  tag scope: Vabc_phase_to_phase_1=global, Voltage_Source_1=global, motor_1=global
  wires:
  Bus Selector/5 -> Gain/1  "<Rotor angle thetam (rad)>"
  pulse 1/1 -> Universal Bridge Inverter 1/1
  Bus Selector/4 -> ωm 1/1  "<Rotor speed wm (rad/s)>"
  Bus Selector/1 -> Bus Creator/1  "<Stator current is_a (A)>"
  Permanent Magnet Synchronous Machine 1/1 -> Bus Selector/1, [motor_1]
  Gain/1 -> theta 1/1
  Bus Creator/1 -> Is abc 1/1
  Bus Selector/3 -> Bus Creator/3  "<Stator current is_c (A)>"
  Bus Selector/2 -> Bus Creator/2  "<Stator current is_b (A)>"
  TLm,1,ref/1 -> Permanent Magnet Synchronous Machine 1/1
  Three-Phase V-I Measurement 1/1 -> [Vabc_phase_to_phase_1]
  Voltage Measurement 1/1 -> Gain1/1
  Gain1/1 -> [Voltage_Source_1]
  connections:
  Permanent Magnet Synchronous Machine 1/LConn2 -- Three-Phase V-I Measurement 1/RConn2
  Permanent Magnet Synchronous Machine 1/LConn1 -- Three-Phase V-I Measurement 1/RConn1
  Permanent Magnet Synchronous Machine 1/LConn3 -- Three-Phase V-I Measurement 1/RConn3
  Universal Bridge Inverter 1/RConn2 -- Voltage Measurement 1/LConn1 -- Vdc 1/LConn1
  Universal Bridge Inverter 1/RConn1 -- Voltage Measurement 1/LConn2 -- Vdc 1/RConn1
  Universal Bridge Inverter 1/LConn1 -- Three-Phase V-I Measurement 1/LConn1
  Universal Bridge Inverter 1/LConn2 -- Three-Phase V-I Measurement 1/LConn2
  Universal Bridge Inverter 1/LConn3 -- Three-Phase V-I Measurement 1/LConn3

== system EDS_Simulink_Model_02/PMSM & Inverter & Energy Source 2 ==
  pulse 2 : Inport
  TLm,2,ref : Inport  Port=2
  Bus Creator : BusCreator  Inputs=3
  Bus Selector : BusSelector  OutputSignals=Stator current is_a (A),Stator current is_b (A),Stator current is_c (A),Rotor speed wm (rad/s),Rotor angle thetam (rad)
  Gain : Gain  Gain=p
  Gain1 : Gain  Gain=-1
  Permanent Magnet Synchronous Machine 2 : spsPermanentMagnetSynchronousMachineLib/Permanent Magnet Synchronous Machine  NbPhases=3  FluxDistribution=Sinusoidal  RotorType=Round  MechanicalLoad=Torque Tm  PresetModel=No  ShowDetailedParameters=on  MeasurementBus=off  Resistance=Rs  Inductance=8.5e-3  dqInductances=[0.005173 0.005507]  La=La  MachineConstant=Torque Constant (N.m / A_peak)  Flux=0.46667  VoltageCst=338.5759  TorqueCst=Kt  Flat=120  Mechanical=[J F p Tf]  PolePairs=4  InitialConditions=[0,0, 0,0]  InitialConditions5ph=[0 0 0 0 0 0]  RefAngle=90 degrees behind phase A axis (modified Park)  IterativeDiscreteModel=Trapezoidal non iterative  TsBlock=-1  TsPowergui=0
  Three-Phase V-I Measurement 2 : spsThreePhaseVIMeasurementLib/Three-Phase V-I Measurement  VoltageMeasurement=phase-to-phase  SetLabelV=off  LabelV=Vabc  Vpu=off  VpuLL=off  CurrentMeasurement=yes  SetLabelI=off  LabelI=Iabc  Ipu=off  Pbase=100e6  Vbase=500e3  OutputType=Complex  PhasorSimulation=off  PSBequivalent=0
  Universal Bridge Inverter 2 : spsUniversalBridgeLib/Universal Bridge  Arms=3  SnubberResistance=R_snubber  SnubberCapacitance=Cs  Device=IGBT / Diodes  Ron=Ron  Lon=0  ForwardVoltages="[Vf  Vfd]"  ForwardVoltage=0  GTOparameters=[ 10e-6 , 20e-6 ]  IGBTparameters=[ 1e-6 , 2e-6 ]  Measurements=Device voltages  Measurements_2=None  converterType=Rectifier
  Vdc 2 : spsDCVoltageSourceLib/DC Voltage Source  Amplitude=Vdc_2  Measurements=None
  Voltage Measurement1 : spsVoltageMeasurementLib/Voltage Measurement  PhasorSimulation=off  OutputType=Complex  PSBequivalent=0
  Is abc 2 : Outport  VectorParamsAs1DForOutWhenUnconnected=off
  theta 2 : Outport  Port=2  VectorParamsAs1DForOutWhenUnconnected=off
  ωm 2 : Outport  Port=3  VectorParamsAs1DForOutWhenUnconnected=off
  tag scope: Vabc_phase_to_phase_2=global, Voltage_Source_2=global, motor_2=global
  wires:
  Bus Selector/5 -> Gain/1  "<Rotor angle thetam (rad)>"
  pulse 2/1 -> Universal Bridge Inverter 2/1
  Bus Selector/4 -> ωm 2/1  "<Rotor speed wm (rad/s)>"
  Bus Selector/1 -> Bus Creator/1  "<Stator current is_a (A)>"
  Permanent Magnet Synchronous Machine 2/1 -> [motor_2], Bus Selector/1
  Gain/1 -> theta 2/1
  Bus Creator/1 -> Is abc 2/1
  Bus Selector/3 -> Bus Creator/3  "<Stator current is_c (A)>"
  Bus Selector/2 -> Bus Creator/2  "<Stator current is_b (A)>"
  TLm,2,ref/1 -> Permanent Magnet Synchronous Machine 2/1
  Three-Phase V-I Measurement 2/1 -> [Vabc_phase_to_phase_2]
  Voltage Measurement1/1 -> Gain1/1
  Gain1/1 -> [Voltage_Source_2]
  connections:
  Permanent Magnet Synchronous Machine 2/LConn2 -- Three-Phase V-I Measurement 2/RConn2
  Permanent Magnet Synchronous Machine 2/LConn1 -- Three-Phase V-I Measurement 2/RConn1
  Permanent Magnet Synchronous Machine 2/LConn3 -- Three-Phase V-I Measurement 2/RConn3
  Universal Bridge Inverter 2/RConn2 -- Voltage Measurement1/LConn1 -- Vdc 2/LConn1
  Universal Bridge Inverter 2/RConn1 -- Vdc 2/RConn1 -- Voltage Measurement1/LConn2
  Universal Bridge Inverter 2/LConn1 -- Three-Phase V-I Measurement 2/LConn1
  Universal Bridge Inverter 2/LConn2 -- Three-Phase V-I Measurement 2/LConn2
  Universal Bridge Inverter 2/LConn3 -- Three-Phase V-I Measurement 2/LConn3

== system EDS_Simulink_Model_02/Pedal ==
  Clock1 : Clock
  Goto1 : Goto  Commented=on  GotoTag=Reference_Speed  TagVisibility=global
  If : If  IfExpression=u1 <= accel_time  ElseIfExpressions="u1 >=  accel_time"  ShowElse=off  ZeroCross=off
  If Action Subsystem : Subsystem  TreatAsAtomicUnit=on
  If Action Subsystem1 : Subsystem  TreatAsAtomicUnit=on
  Merge : Merge
  Sum7 : Sum  Commented=on  Inputs=|++
  w ref pedal potision 1 : Step  Commented=on  Time=time_w_ref_1  Before=w_ref_initial  After=w_ref_1  SampleTime=0
  w ref pedal potision 2 : Step  Commented=on  Time=time_w_ref_2  After=-w_ref_1+w_ref_2  SampleTime=0
  reference speed ωref : Outport
  tag scope: Reference_Speed=global
  wires:
  w ref pedal potision 2/1 -> Sum7/2
  w ref pedal potision 1/1 -> Sum7/1  "w ref"
  Sum7/1 -> Goto1/1  "w ref"
  Clock1/1 -> If/1
  If/1 -> If Action Subsystem/Action
  If/2 -> If Action Subsystem1/Action
  If Action Subsystem/1(Out1) -> Merge/1
  If Action Subsystem1/1(Out1) -> Merge/2
  Merge/1 -> reference speed ωref/1, [Reference_Speed]

== system EDS_Simulink_Model_02/Plots 1&2 ==
  " Plots Motor 1" : Subsystem  Commented=on
  Current 1 & 2 : Subsystem
  EDS : Subsystem
  Plots Motor 2 : Subsystem  Commented=on
  SVPWM 1 & 2 : Subsystem
  Speed 1 & 2 : Subsystem
  Torque 1 & 2 : Subsystem
  Voltage 1 & 2 : Subsystem

== system EDS_Simulink_Model_02/Reference Torque Calculation 1 ==
  ωw,1,ref : Inport
  K7 : Gain  Gain=1/(n_eff_gear*i_gear)
  Load Wheel Torque Calculation 1 : MATLAB Function  TreatAsAtomicUnit=on
  TLm,1,ref : Outport
  tag scope: Ref_Load_Motor_Torque_1=global, Ref_Load_Wheel_Torque_1=global
  wires:
  Load Wheel Torque Calculation 1/1(Tw1) -> [Ref_Load_Wheel_Torque_1], K7/1  "ref load wheel torque TLw,1,ref"
  K7/1 -> TLm,1,ref/1, [Ref_Load_Motor_Torque_1]  "ref load motor torque TLm,1,ref"
  ωw,1,ref/1 -> Load Wheel Torque Calculation 1/1(w1)  "ref wheel speed 1: ωw,1,ref"

== system EDS_Simulink_Model_02/Reference Torque Calculation 2 ==
  ωw,2,ref : Inport
  K8 : Gain  Gain=1/(n_eff_gear*i_gear)
  Load Wheel Torque Calculation 2 : MATLAB Function  TreatAsAtomicUnit=on
  TLm,2,ref : Outport
  tag scope: Ref_Load_Motor_Torque_2=global, Ref_Load_Wheel_Torque_2=global
  wires:
  Load Wheel Torque Calculation 2/1(Tw2) -> [Ref_Load_Wheel_Torque_2], K8/1  "ref load wheel torque TLw,2,ref"
  ωw,2,ref/1 -> Load Wheel Torque Calculation 2/1(w2)  "ref wheel speed 2: ωw,2,ref"
  K8/1 -> [Ref_Load_Motor_Torque_2], TLm,2,ref/1  "ref load motor torque TLm,2,ref"

== system EDS_Simulink_Model_02/Steering Subsystem ==
  Sum2 : Sum  Inputs=|++++
  steering angle 1 : Step  Time=time_steering_angle_1  Before=steering_angle_initial  After=steering_angle_1  SampleTime=0
  steering angle 2 : Step  Time=time_steering_angle_2  After=-steering_angle_1+steering_angle_2  SampleTime=0
  steering angle 3 : Step  Time=time_steering_angle_3  After=-steering_angle_2+steering_angle_3  SampleTime=0
  steering angle 4 : Step  Time=time_steering_angle_4  After=-steering_angle_3+steering_angle_4  SampleTime=0
  steering angle : Outport
  tag scope: Steering_Angle=global
  wires:
  Sum2/1 -> [Steering_Angle], steering angle/1
  steering angle 1/1 -> Sum2/1
  steering angle 2/1 -> Sum2/2
  steering angle 3/1 -> Sum2/3
  steering angle 4/1 -> Sum2/4

== system EDS_Simulink_Model_02/Subsystem Gearbox - Wheel 1 (Left) ==
  motor speed 1 : Inport
  Gearbox 1 : MATLAB Function  TreatAsAtomicUnit=on
  Wheel Torque Calculation 1 : MATLAB Function  TreatAsAtomicUnit=on
  tag scope: Load_Wheel_Torque_1=global, Wheel_Speed_1=global
  wires:
  Gearbox 1/1(w_speed_1) -> Wheel Torque Calculation 1/1(w1), [Wheel_Speed_1]
  Wheel Torque Calculation 1/1(Tw1) -> [Load_Wheel_Torque_1]
  motor speed 1/1 -> Gearbox 1/1(m_speed_1)

== system EDS_Simulink_Model_02/Subsystem Gearbox - Wheel 2 (Right) ==
  motor speed 2 : Inport
  Gearbox 2 : MATLAB Function  TreatAsAtomicUnit=on
  Wheel Torque Calculation 2 : MATLAB Function  TreatAsAtomicUnit=on
  tag scope: Load_Wheel_Torque_2=global, Wheel_Speed_2=global
  wires:
  Gearbox 2/1(w_speed_2) -> [Wheel_Speed_2], Wheel Torque Calculation 2/1(w2)
  Wheel Torque Calculation 2/1(Tw2) -> [Load_Wheel_Torque_2]
  motor speed 2/1 -> Gearbox 2/1(m_speed_2)

== system EDS_Simulink_Model_02/Control Systetm 1 (FOC & SVPWM)/Clark Transformation 1 ==
  I_abc : Inport
  " " : Fcn  Expr=sqrt(3)/2*(u[2]-u[3]) * sqrt(2/3)
  " " : Fcn  Expr=(u[1]-0.5*(u[2]+u[3])) * sqrt(2/3)
  Mux : Mux  Inputs=[3]
  I_alpha : Outport  InitialOutput=0  VectorParamsAs1DForOutWhenUnconnected=off
  I_beta : Outport  Port=2  InitialOutput=0  VectorParamsAs1DForOutWhenUnconnected=off
  tag scope: I_alpha_1=global, I_beta_1=global
  wires:
  " "/1 -> [I_beta_1], I_beta/1
  " "/1 -> [I_alpha_1], I_alpha/1
  Mux/1 -> " "/1, " "/1
  I_abc/1 -> Mux/1

== system EDS_Simulink_Model_02/Control Systetm 1 (FOC & SVPWM)/Park Inverse Transformation 1  ==
  Vq : Inport
  Vd : Inport  Port=2
  theta : Inport  Port=3
  Fcn : Fcn  Expr=u(1)*cos(u(3)) + u(2)*sin(u(3))
  Fcn1 : Fcn  Expr=u(1)*cos(u(3)-2*pi/3) + u(2)*sin(u(3)-2*pi/3)
  Fcn2 : Fcn  Expr=u(1)*cos(u(3)+2*pi/3) + u(2)*sin(u(3)+2*pi/3)
  Gain1 : Gain  Gain=1/sqrt(3)  SaturateOnIntegerOverflow=on  OutDataTypeStr=Inherit: Same as input  ParamDataTypeStr=Inherit: Same as input
  Mux : Mux  Inputs=3
  Mux1 : Mux  Inputs=3
  Mux2 : Mux  Inputs=[3]
  i_alpha : Fcn  Expr=u[1]
  i_beta : Fcn  Expr=u[1]+2*u[2]
  Valpha : Outport  InitialOutput=0  VectorParamsAs1DForOutWhenUnconnected=off
  Vbeta : Outport  Port=2  InitialOutput=0  VectorParamsAs1DForOutWhenUnconnected=off
  wires:
  Fcn/1 -> Mux1/1
  Vd/1 -> Mux/2
  Fcn2/1 -> Mux1/3
  Fcn1/1 -> Mux1/2
  Mux/1 -> Fcn1/1, Fcn2/1, Fcn/1
  Vq/1 -> Mux/1
  theta/1 -> Mux/3
  Mux2/1 -> i_alpha/1, i_beta/1
  i_beta/1 -> Gain1/1
  i_alpha/1 -> Valpha/1
  Gain1/1 -> Vbeta/1
  Mux1/1 -> Mux2/1

== system EDS_Simulink_Model_02/Control Systetm 1 (FOC & SVPWM)/Plark Transformation 1 ==
  I_alpha : Inport
  I_beta : Inport  Port=2
  Theta : Inport  Port=3
  " " : Fcn  Expr=-u[2]*u[3]+u[1]*u[4]
  " " : Fcn  Expr=u[1]*u[3]+u[2]*u[4]
  Fcn : Fcn  Expr=sin(u)
  Fcn1 : Fcn  Expr=cos(u)
  Mux : Mux  Inputs=[1 1 1 1]
  Id : Outport  InitialOutput=0  VectorParamsAs1DForOutWhenUnconnected=off
  Iq : Outport  Port=2  InitialOutput=0  VectorParamsAs1DForOutWhenUnconnected=off
  wires:
  Fcn/1 -> Mux/2
  Fcn1/1 -> Mux/1
  Mux/1 -> " "/1, " "/1
  I_alpha/1 -> Mux/3
  I_beta/1 -> Mux/4
  Theta/1 -> Fcn1/1, Fcn/1
  " "/1 -> Id/1
  " "/1 -> Iq/1

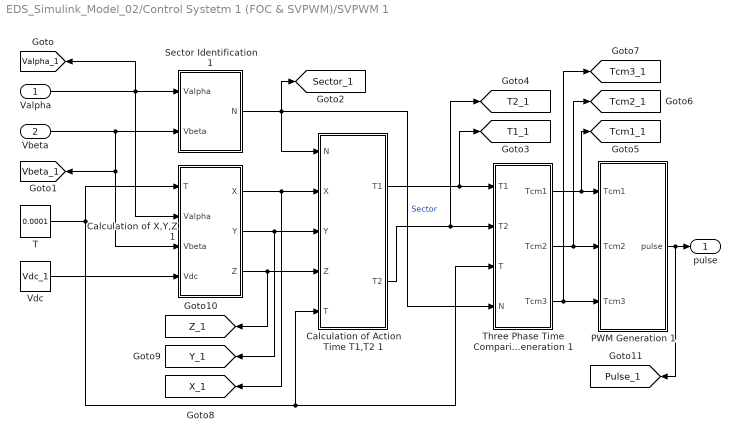
== system EDS_Simulink_Model_02/Control Systetm 1 (FOC & SVPWM)/SVPWM 1 ==
  Valpha : Inport
  Vbeta : Inport  Port=2
  Calculation of Action Time T1,T2 1 : Subsystem
  Calculation of X,Y,Z 1 : Subsystem
  PWM Generation 1 : Subsystem
  Sector Identification 1 : Subsystem
  T : Constant  Value=0.0001
  Three Phase Time Comparison Generation 1 : Subsystem
  Vdc : Constant  Value=Vdc_1
  pulse : Outport  VectorParamsAs1DForOutWhenUnconnected=off
  tag scope: Pulse_1=global, Sector_1=global, T1_1=global, T2_1=global, Tcm1_1=global, Tcm2_1=global, Tcm3_1=global, Valpha_1=global, Vbeta_1=global, X_1=global, Y_1=global, Z_1=global
  wires:
  T/1 -> Three Phase Time Comparison Generation 1/3(T), Calculation of Action Time T1,T2 1/5(T), Calculation of X,Y,Z 1/1(T)
  Vdc/1 -> Calculation of X,Y,Z 1/4(Vdc)
  Sector Identification 1/1(N) -> Calculation of Action Time T1,T2 1/1(N), Three Phase Time Comparison Generation 1/4(N), [Sector_1]  "Sector"
  Calculation of X,Y,Z 1/1(X) -> Calculation of Action Time T1,T2 1/2(X), [X_1]
  Calculation of X,Y,Z 1/2(Y) -> Calculation of Action Time T1,T2 1/3(Y), [Y_1]
  Calculation of X,Y,Z 1/3(Z) -> Calculation of Action Time T1,T2 1/4(Z), [Z_1]
  Three Phase Time Comparison Generation 1/1(Tcm1) -> [Tcm1_1], PWM Generation 1/1(Tcm1)
  Three Phase Time Comparison Generation 1/2(Tcm2) -> [Tcm2_1], PWM Generation 1/2(Tcm2)
  Three Phase Time Comparison Generation 1/3(Tcm3) -> [Tcm3_1], PWM Generation 1/3(Tcm3)
  Valpha/1 -> [Valpha_1], Sector Identification 1/1(Valpha), Calculation of X,Y,Z 1/2(Valpha)
  Calculation of Action Time T1,T2 1/1(T1) -> [T1_1], Three Phase Time Comparison Generation 1/1(T1)
  Calculation of Action Time T1,T2 1/2(T2) -> Three Phase Time Comparison Generation 1/2(T2), [T2_1]
  Vbeta/1 -> [Vbeta_1], Calculation of X,Y,Z 1/3(Vbeta), Sector Identification 1/2(Vbeta)
  PWM Generation 1/1(pulse) -> [Pulse_1], pulse/1

== system EDS_Simulink_Model_02/Control Systetm 2 (FOC & SVPWM)/Clark Transformation 2 ==
  Is_abc : Inport
  " " : Fcn  Expr=sqrt(3)/2*(u[2]-u[3]) * sqrt(2/3)
  " " : Fcn  Expr=(u[1]-0.5*(u[2]+u[3])) * sqrt(2/3)
  MATLAB Function : MATLAB Function  Commented=on  TreatAsAtomicUnit=on
  MATLAB Function1 : MATLAB Function  Commented=on  TreatAsAtomicUnit=on
  Mux : Mux  Inputs=[3]
  Mux2 : Mux  Commented=on  Inputs=[3]
  I_alpha : Outport  InitialOutput=0  VectorParamsAs1DForOutWhenUnconnected=off
  I_beta : Outport  Port=2  InitialOutput=0  VectorParamsAs1DForOutWhenUnconnected=off
  tag scope: I_alpha_2=global, I_beta_2=global
  wires:
  " "/1 -> [I_beta_2], I_beta/1
  MATLAB Function/1(y) -> ?
  MATLAB Function1/1(y) -> ?
  ? -> Mux2/1
  Mux2/1 -> MATLAB Function1/1(u), MATLAB Function/1(u)
  " "/1 -> [I_alpha_2], I_alpha/1
  Mux/1 -> " "/1, " "/1
  Is_abc/1 -> Mux/1

== system EDS_Simulink_Model_02/Control Systetm 2 (FOC & SVPWM)/Park Inverse Transformation 2  ==
  Vq : Inport
  Vd : Inport  Port=2
  theta : Inport  Port=3
  Fcn : Fcn  Expr=u(1)*cos(u(3)) + u(2)*sin(u(3))
  Fcn1 : Fcn  Expr=u(1)*cos(u(3)-2*pi/3) + u(2)*sin(u(3)-2*pi/3)
  Fcn2 : Fcn  Expr=u(1)*cos(u(3)+2*pi/3) + u(2)*sin(u(3)+2*pi/3)
  Gain1 : Gain  Gain=1/sqrt(3)  SaturateOnIntegerOverflow=on  OutDataTypeStr=Inherit: Same as input  ParamDataTypeStr=Inherit: Same as input
  Mux : Mux  Inputs=3
  Mux1 : Mux  Inputs=3
  Mux2 : Mux  Inputs=[3]
  i_alpha : Fcn  Expr=u[1]
  i_beta : Fcn  Expr=u[1]+2*u[2]
  Valpha : Outport  InitialOutput=0  VectorParamsAs1DForOutWhenUnconnected=off
  Vbeta : Outport  Port=2  InitialOutput=0  VectorParamsAs1DForOutWhenUnconnected=off
  wires:
  Fcn/1 -> Mux1/1
  Vd/1 -> Mux/2
  Fcn2/1 -> Mux1/3
  Fcn1/1 -> Mux1/2
  Mux/1 -> Fcn1/1, Fcn2/1, Fcn/1
  Vq/1 -> Mux/1
  theta/1 -> Mux/3
  Mux2/1 -> i_alpha/1, i_beta/1
  i_beta/1 -> Gain1/1
  i_alpha/1 -> Valpha/1
  Gain1/1 -> Vbeta/1
  Mux1/1 -> Mux2/1

== system EDS_Simulink_Model_02/Control Systetm 2 (FOC & SVPWM)/Plark Transformation 2 ==
  I_alpha : Inport
  I_beta : Inport  Port=2
  Theta : Inport  Port=3
  " " : Fcn  Expr=-u[2]*u[3]+u[1]*u[4]
  " " : Fcn  Expr=u[1]*u[3]+u[2]*u[4]
  Fcn : Fcn  Expr=sin(u)
  Fcn1 : Fcn  Expr=cos(u)
  Mux : Mux  Inputs=[1 1 1 1]
  Id : Outport  InitialOutput=0  VectorParamsAs1DForOutWhenUnconnected=off
  Iq : Outport  Port=2  InitialOutput=0  VectorParamsAs1DForOutWhenUnconnected=off
  wires:
  Fcn/1 -> Mux/2
  Fcn1/1 -> Mux/1
  Mux/1 -> " "/1, " "/1
  I_alpha/1 -> Mux/3
  I_beta/1 -> Mux/4
  Theta/1 -> Fcn1/1, Fcn/1
  " "/1 -> Id/1
  " "/1 -> Iq/1

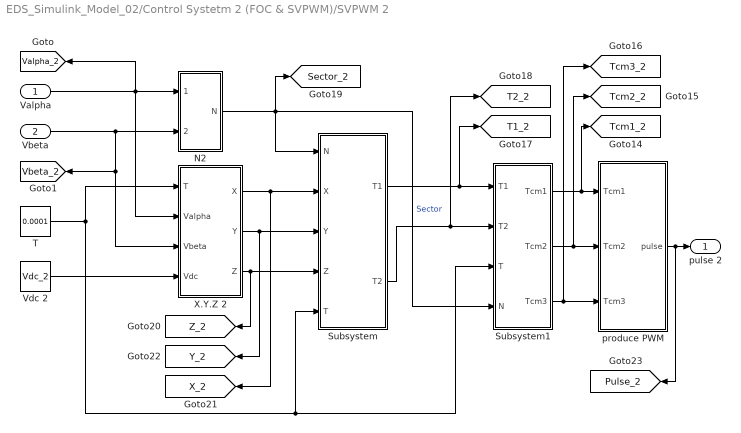
== system EDS_Simulink_Model_02/Control Systetm 2 (FOC & SVPWM)/SVPWM 2 ==
  Valpha : Inport
  Vbeta : Inport  Port=2
  N2 : Subsystem
  Subsystem : Subsystem
  Subsystem1 : Subsystem
  T : Constant  Value=0.0001
  Vdc 2 : Constant  Value=Vdc_2
  X.Y.Z 2 : Subsystem
  produce PWM : Subsystem
  pulse 2 : Outport  VectorParamsAs1DForOutWhenUnconnected=off
  tag scope: Pulse_2=global, Sector_2=global, T1_2=global, T2_2=global, Tcm1_2=global, Tcm2_2=global, Tcm3_2=global, Valpha_2=global, Vbeta_2=global, X_2=global, Y_2=global, Z_2=global
  wires:
  T/1 -> Subsystem/5(T), Subsystem1/3(T), X.Y.Z 2/1(T)
  Vdc 2/1 -> X.Y.Z 2/4(Vdc)
  Valpha/1 -> [Valpha_2], N2/1(Valpha), X.Y.Z 2/2(Valpha)
  Vbeta/1 -> [Vbeta_2], X.Y.Z 2/3(Vbeta), N2/2(Vbeta)
  Subsystem1/2(Tcm2) -> [Tcm2_2], produce PWM/2(Tcm2)
  Subsystem1/1(Tcm1) -> [Tcm1_2], produce PWM/1(Tcm1)
  Subsystem1/3(Tcm3) -> [Tcm3_2], produce PWM/3(Tcm3)
  Subsystem/2(T2) -> [T2_2], Subsystem1/2(T2)
  Subsystem/1(T1) -> [T1_2], Subsystem1/1(T1)
  N2/1(N) -> Subsystem1/4(N), Subsystem/1(N), [Sector_2]  "Sector"
  X.Y.Z 2/3(Z) -> [Z_2], Subsystem/4(Z)
  X.Y.Z 2/2(Y) -> [Y_2], Subsystem/3(Y)
  X.Y.Z 2/1(X) -> [X_2], Subsystem/2(X)
  produce PWM/1(pulse) -> [Pulse_2], pulse 2/1

== system EDS_Simulink_Model_02/Pedal/If Action Subsystem ==
  Action Port : ActionPort  ActionPortLabel=if(u1 <= accel_time)
  Clock : Clock
      settings: Decimation=5
  fun3 : MATLAB Function  TreatAsAtomicUnit=on
  Out1 : Outport
  wires:
  fun3/1(y) -> Out1/1
  Clock/1 -> fun3/1(x)

== system EDS_Simulink_Model_02/Pedal/If Action Subsystem1 ==
  Action Port : ActionPort  ActionPortLabel="elseif(u1 >=  accel_time)"
  fun3 : MATLAB Function  TreatAsAtomicUnit=on
  Out1 : Outport
  wires:
  fun3/1(y) -> Out1/1
